simulink model "func3_c"  (R2023a)
settings: Solver=VariableStepAuto  StartTime=0.0  StopTime=10.0  RelTol=1e-3  EnableMultiTasking=on
libraries: vmcUtilities x2, templatized_input_3_lib x1
settings Model: Creator=abehbood  LastModifiedBy=robg
settings SolverCC: AlgebraicLoopSolver=TrustRegion
settings DataIOCC: ReturnWorkspaceOutputs=off
settings OptimizationCC: LifeSpan=inf
settings DebuggingCC: UnconnectedInputMsg=warning  UnconnectedOutputMsg=warning  UnconnectedLineMsg=warning  SFUnexpectedBacktrackingDiag=warning  SFNoUnconditionalDefaultTransitionDiag=warning  ArithmeticOperatorsInVariantConditions=warning
settings ModelReferenceCC: EnableRefExpFcnMdlSchedulingChecks=on
settings SFSimCC: SimUseLocalCustomCode=off  CustomCodeUndefinedFunction=UseInterfaceOnly
settings RTWCC: RTWUseLocalCustomCode=off  DLArmComputeVersion=19.05
settings CodeAppCC: StateflowObjectComments=on
settings GRTTargetCC: TargetLangStandard=C89/C90 (ANSI)
settings ConfigComp: CovMetricSettings=dw  CovSaveCumulativeToWorkspaceVar=on  CovSaveSingleToWorkspaceVar=on  CovExternalEMLEnable=off

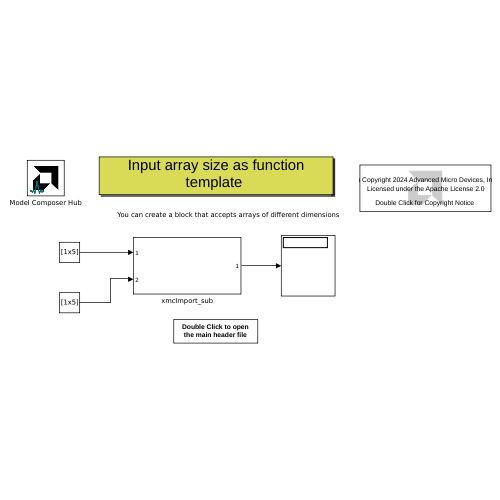
[thumbnail: Simulink's stored preview of the top-level diagram]
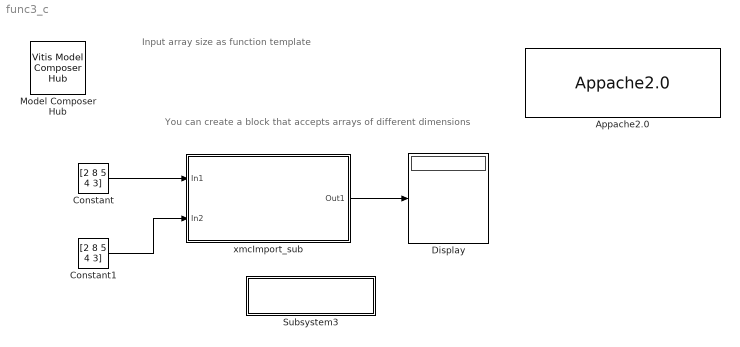
== system func3_c ==
  note: You can create a block that accepts arrays of different dimensions
  note: Input array size as function template
  Appache2.0 : vmcUtilities/Appache2.0
  Constant : Constant  Value=[2 8 5 4 3]  OutDataTypeStr=int16  SampleTime=1
  Constant1 : Constant  Value=[2 8 5 4 3]  OutDataTypeStr=int16  SampleTime=1
  Display : Display
  Model Composer Hub : vmcUtilities/Vitis Model Composer Hub  Tag=genX  CodeGeneration=off  SubsystemName=xmcImport_sub  StartColumn=1  NumberOfColumns=1  TargetDirectory=./code  exportDesign=off  analyzeDesign=off  validateDesignOnHw=off  ExportType=IP Catalog  IpVendor=xilinx.com  IpLibrary=hls  IpVersion=1.0  IpHWLanguage=Verilog  AieCompilerOptions={}  AieSimulatorOptions={}  CreateTestbench=off  TestbenchStackSize=10  RunRtlSim=off  RunCSim=off  RunAieSim=off  AieSimTimeout=50000  RunAieSimProfiling=off  LaunchVitisAnalyzer=off  PlotOutput=off  RunX86Sim=off  X86SimTimeout=10  GenHwImage=off  GenLibadfXo=off  GenHwValidationCode=off  PlatformType=Not Specified  HwSystemType=Baremetal  HwValidationTarget=hw  ProjDevice=xcku11p-ffva1156-1-e  ProjDevicePart=xcku11p-ffva1156-1-e  SamplePeriod=-1  ClockFrequency=200  DataPathParallelism=1  xilinxfamily=Kintex7  part=xc7k325t  speed=-3  package=fbg676  directory=./netlist  testbench=off  incr_netlist=off  synthesis_tool=Vivado  clock_wrapper=Clock Enables  dbl_ovrd=According to Block Masks  dcm_input_clock_period=10  sysclk_period=10  simulink_period=1  eval_field=0  LogFileName=''  NThreads=4
  Subsystem3 : Subsystem
      settings: OpenFcn=xmcOpenFileEx
      mask Display: disp(sprintf('Double Click to open\nthe main header file'))
  xmcImport_sub : Subsystem
  wires:
  Constant/1 -> xmcImport_sub/1(In1)
  Constant1/1 -> xmcImport_sub/2(In2)
  xmcImport_sub/1(Out1) -> Display/1

== system func3_c/Subsystem3 ==

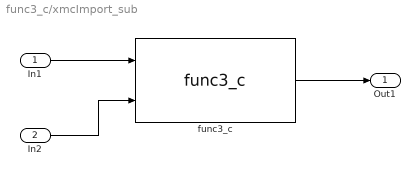
== system func3_c/xmcImport_sub ==
  In1 : Inport
  In2 : Inport  Port=2
  func3_c : templatized_input_3_lib/func3_c  LibraryFunction=func3_c  IncludeFiles={'func3_c.h'}  SourceFiles={}  IncludeDirectories={}  TemplateParams={'int SIZE'}  FunctionParamTypes={xmcDataType('void'); xmcDataType('const int16_t'); xmcDataType('const int16_t'); xmcDataType('int16_t')}  FunctionParamPassbys={0.000000000000000000e+00; 0.000000000000000000e+00; 0.000000000000000000e+00; 0.000000000000000000e+00}  FunctionParamDimensions={'1'; '[SIZE]'; '[SIZE]'; '[SIZE]'}  FunctionParamNames={'return'; 'in1'; 'in2'; 'out'}  FunctionParamDir={0.000000000000000000e+00; 1.000000000000000000e+00; 1.000000000000000000e+00; 2.000000000000000000e+00}  FunctionParamSupportsStreaming={false; false; false; false}  BufferDepth={'0'}  FunctionParamValues={'0'; '0'; '0'; '0'}  ThroughputFactors={''}
  Out1 : Outport
  wires:
  In2/1 -> func3_c/2
  func3_c/1 -> Out1/1
  In1/1 -> func3_c/1
